simulink model "Task_02_Sim"  (R2024a)
settings: Solver=VariableStepAuto  StartTime=0.0  StopTime=40.0  RelTol=1e-3
settings Model: Creator=PMYLS  LastModifiedBy=PMYLS

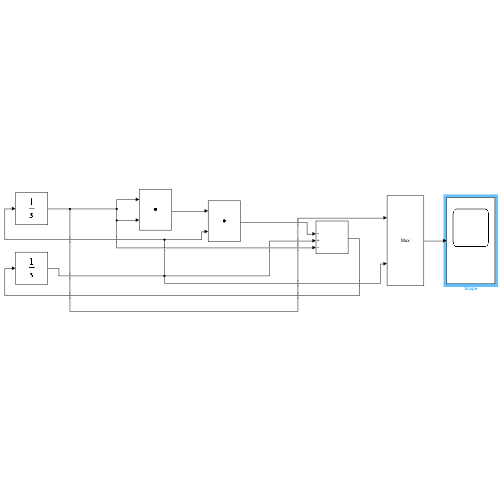
[thumbnail: Simulink's stored preview of the top-level diagram]
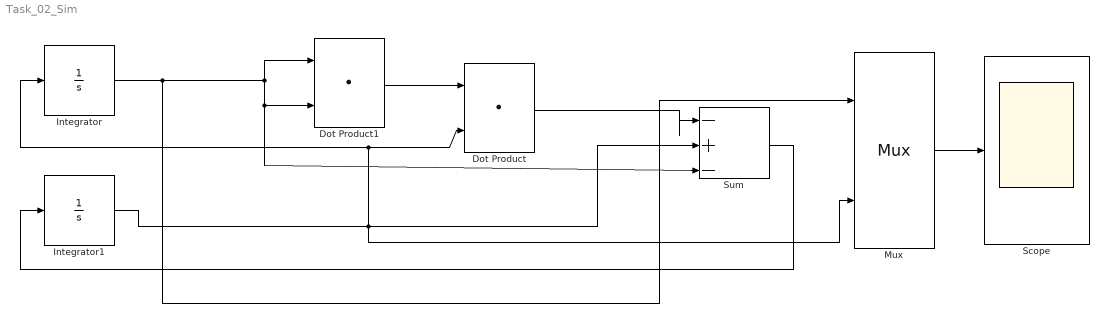
== system Task_02_Sim ==
  Dot Product : DotProduct  OutDataTypeStr=Inherit: Inherit via internal rule
  Dot Product1 : DotProduct  OutDataTypeStr=Inherit: Inherit via internal rule
  Integrator : Integrator
  Integrator1 : Integrator  InitialCondition=1
  Mux : Mux  Inputs=2
  Scope : Scope
  Sum : Sum  Inputs=|-+-
  wires:
  Mux/1 -> Scope/1
  Dot Product1/1 -> Dot Product/1
  Integrator/1 -> Mux/1, Dot Product1/2, Sum/3, Dot Product1/1
  Integrator1/1 -> Dot Product/2, Integrator/1, Mux/2, Sum/2
  Sum/1 -> Integrator1/1
  Dot Product/1 -> Sum/1
